simulink model "A1"  (R2024a)
settings: Solver=ode45  StartTime=0.0  StopTime=10  FixedStep=0.001  RelTol=1e-3
values from neighbouring files (symbols this model uses):
  a = 5    [A1_mat.m]
  b = 0.01    [A1_mat.m]
  c = 3    [A1_mat.m]
  d = 0.0001    [A1_mat.m]
settings Model: Creator=Flipper  LastModifiedBy=Flipper

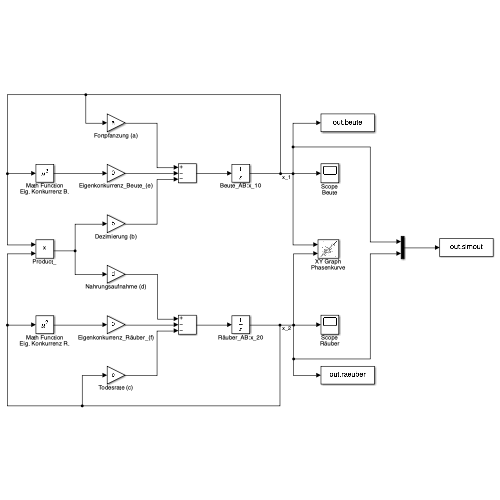
[thumbnail: Simulink's stored preview of the top-level diagram]
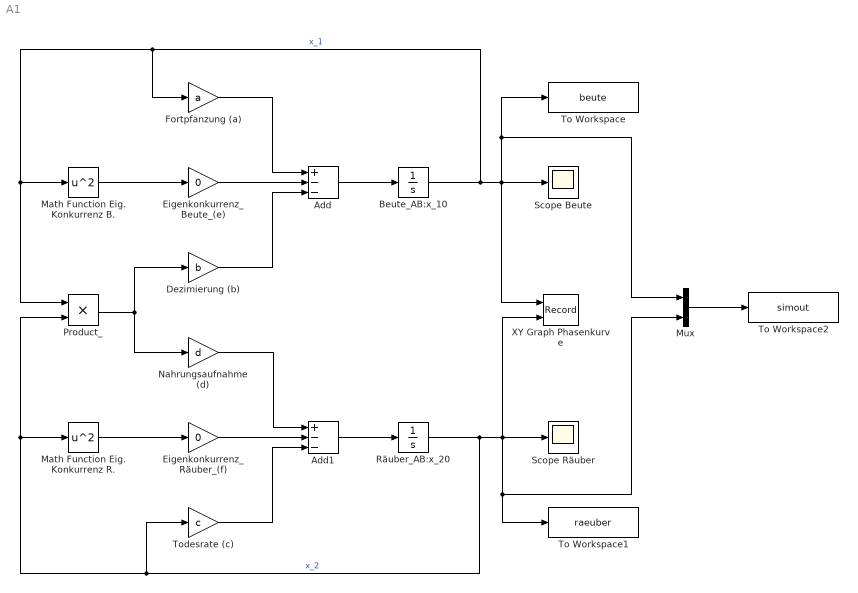
== system A1 ==
  Add : Sum  Inputs=+--
  Add1 : Sum  Inputs=+--
  Beute_AB:x_10 : Integrator  InitialCondition=30000
  Dezimierung (b) : Gain  Gain=b
  Eigenkonkurrenz_Beute_(e) : Gain  Gain=0
  Eigenkonkurrenz_Räuber_(f) : Gain  Gain=0
  Fortpfanzung (a) : Gain  Gain=a
  Math Function Eig. Konkurrenz B. : Math  Operator=square
  Math Function Eig. Konkurrenz R. : Math  Operator=square
  Mux : Mux  Inputs=2
  Nahrungsaufnahme (d) : Gain  Gain=d
  Product_ : Product
  Räuber_AB:x_20 : Integrator  InitialCondition=1000
  Scope Beute : Scope
  Scope Räuber : Scope
  To Workspace : ToWorkspace  VariableName=beute  SaveFormat=Timeseries  SampleTime=-1
  To Workspace1 : ToWorkspace  VariableName=raeuber  SaveFormat=Timeseries  SampleTime=-1
  To Workspace2 : ToWorkspace  VariableName=simout  SaveFormat=Timeseries  SampleTime=-1
  Todesrate (c) : Gain  Gain=c
  XY Graph Phasenkurve : Record  FileSettingsInternal="{\"entries\":[{\"content\":{\"excelSettings\":{\"content\":{},\"type\":\"Streamout.ExcelSettings\"}},\"type\":\"Streamout.FileSettingStorage\",\"uuid\":\"\"}],\"packageUris\":[\"http:\\/\\/schema.mathworks.com\\/mf0\\/streamout_blocks\\/R2020a\"],\"version\":\"1.0\"}"  Layout=[1 1]  SignalsInternal="{\"entries\":[{\"content\":{\"signals\":[{\"content\":{\"blockPath\":[],\"dimensions\":[1],\"domain\":\"\",\"lineColor\":\"#a2142f\",\"plots\":[ 1 ],\"port\":1,\"sid\":[\"\"],\"signalID\":1,\"signalName\":\"x_1\"},\"type\":\"RecordBlkView.Signal\",\"uuid\":\"\"},{\"content\":{\"blockPath\":[],\"dimensions\":[1],\"domain\":\"\",\"lineColor\":\"#139fff\",\"plots\":[ 1 ],\"port\":2,\"sid\":[\"\"],\"signalID\":2,\"signalName\":\"x_2\"},\"type\":\"RecordBlkView.Signal\",\"uuid\":\"\"}]},\"type\":\"RecordBlkView.InputSignals\",\"uuid\":\"\"}],\"packageUris\":[\"http:\\/\\/schema.mathworks.com\\/mf0\\/streamout_blocks\\/R2020a\"],\"version\":\"1.0\"}"  VisualizationBindings="{\"xyplotplugin\":{\"info\":[{\"series\":[{\"bindingParametersList\":[{\"parameter\":\"X-Axis\",\"signalID\":1,\"signalName\":\"x_1\"},{\"parameter\":\"Y-Axis\",\"signalID\":2,\"signalName\":\"x_2\"}],\"seriesID\":0}],\"subplotID\":1}]}}"  CompatibilityTag=XY
  wires:
  Math Function Eig. Konkurrenz B./1 -> Eigenkonkurrenz_Beute_(e)/1
  Product_/1 -> Nahrungsaufnahme (d)/1, Dezimierung (b)/1
  Math Function Eig. Konkurrenz R./1 -> Eigenkonkurrenz_Räuber_(f)/1
  Eigenkonkurrenz_Beute_(e)/1 -> Add/2
  Dezimierung (b)/1 -> Add/3
  Nahrungsaufnahme (d)/1 -> Add1/1
  Eigenkonkurrenz_Räuber_(f)/1 -> Add1/2
  Todesrate (c)/1 -> Add1/3
  Fortpfanzung (a)/1 -> Add/1
  Add/1 -> Beute_AB:x_10/1
  Beute_AB:x_10/1 -> Fortpfanzung (a)/1, Product_/1, Math Function Eig. Konkurrenz B./1, Mux/1, To Workspace/1, XY Graph Phasenkurve/1, Scope Beute/1  "x_1"
  Add1/1 -> Räuber_AB:x_20/1
  Räuber_AB:x_20/1 -> Todesrate (c)/1, Product_/2, Math Function Eig. Konkurrenz R./1, Mux/2, To Workspace1/1, XY Graph Phasenkurve/2, Scope Räuber/1  "x_2"
  Mux/1 -> To Workspace2/1
